simulink model "Lab3_sol"  (R2024a)
settings: Solver=VariableStepAuto  StartTime=0.0  StopTime=10000  MaxStep=0.1  RelTol=1e-3
values from neighbouring files (symbols this model uses):
  A = [-P1 0 -Gb;0 -n 0;0 P3 -P2]    [Bergman_param.m]
  B = [0 1/Vg;1/V1 0;0 0]    [Bergman_param.m]
  Gb = 81    [Bergman_param.m]
  Ib = 15    [Bergman_param.m]
  n = 5/54    (= 0.0925925925926)    [Bergman_param.m]
  p1 = P1    (= 0.003)    [Bergman_param.m]
  p2 = P2    (= 0.025)    [Bergman_param.m]
  p3 = P3    (= 1.3e-05)    [Bergman_param.m]
  V1 = 12    [Bergman_param.m]
undefined symbols (not defined in the file or in its folder): r_, VG
libraries: simulink x4
settings Model: Creator=Diego Regruto  LastModifiedBy=luigi
settings RTWCC: GPUComputeCapability=3.5

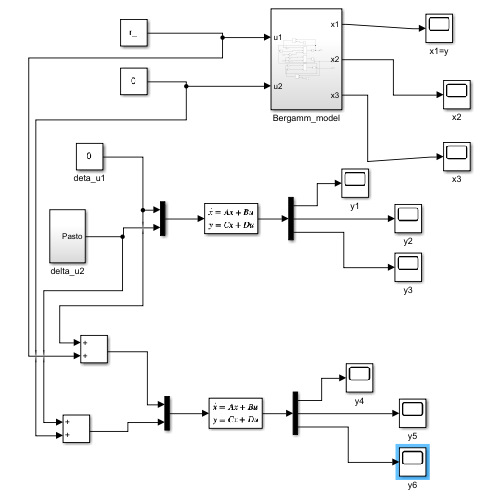
[thumbnail: Simulink's stored preview of the top-level diagram]
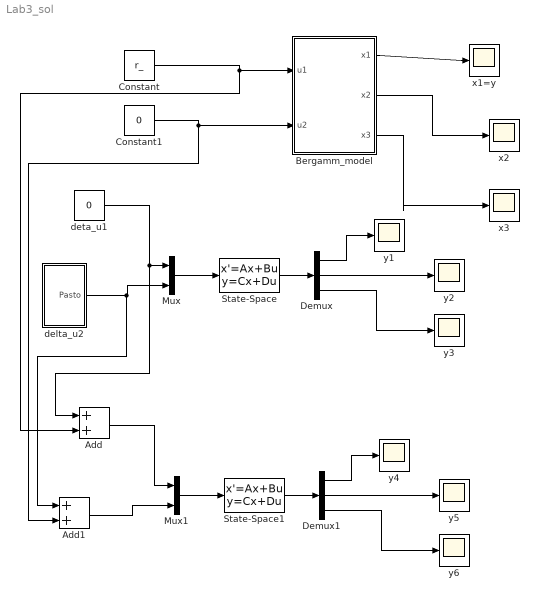
== system Lab3_sol ==
  Add : Sum
  Add1 : Sum
  Bergamm_model : Subsystem
  Constant : Constant  Value=r_
  Constant1 : Constant  Value=0
  Demux : Demux  Outputs=3
  Demux1 : Demux  Outputs=3
  Mux : Mux  Inputs=2
  Mux1 : Mux  Inputs=2
  State-Space : StateSpace  A=A  B=B  C=eye(3,3)  D=zeros(3,2)  InitialCondition=[9 0 0]'
  State-Space1 : StateSpace  A=A  B=B  C=eye(3,3)  D=zeros(3,2)  InitialCondition=[9+81 15 0]'
  delta_u2 : Subsystem
  deta_u1 : Constant  Value=0
  x1=y : Scope
  x2 : Scope
  x3 : Scope
  y{1..6} (6 alike) : Scope
  wires:
  Constant/1 -> Add/2, Bergamm_model/1(u1)
  Constant1/1 -> Add1/2, Bergamm_model/2(u2)
  Bergamm_model/1(x1) -> x1=y/1
  Bergamm_model/2(x2) -> x2/1
  Bergamm_model/3(x3) -> x3/1
  State-Space/1 -> Demux/1
  Mux/1 -> State-Space/1
  Demux/1 -> y1/1
  Demux/2 -> y2/1
  Demux/3 -> y3/1
  delta_u2/1(Pasto) -> Add1/1, Mux/2
  deta_u1/1 -> Add/1, Mux/1
  Demux1/3 -> y6/1
  Mux1/1 -> State-Space1/1
  State-Space1/1 -> Demux1/1
  Demux1/1 -> y4/1
  Add1/1 -> Mux1/2
  Demux1/2 -> y5/1
  Add/1 -> Mux1/1

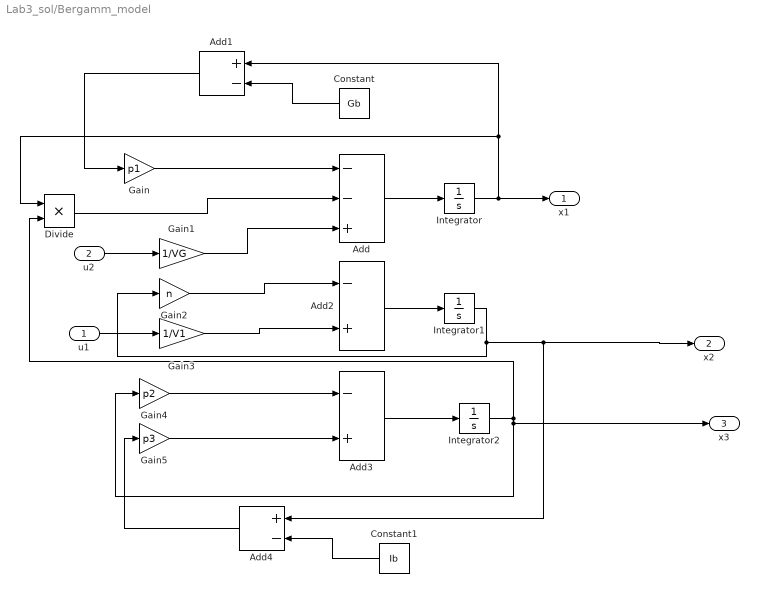
== system Lab3_sol/Bergamm_model ==
  u1 : Inport
  u2 : Inport  Port=2
  Add : Sum  Inputs=--+
  Add1 : Sum  Inputs=+-
  Add2 : Sum  Inputs=-+
  Add3 : Sum  Inputs=-+
  Add4 : Sum  Inputs=+-
  Constant : Constant  Value=Gb
  Constant1 : Constant  Value=Ib
  Divide : Product  Inputs=**
  Gain : Gain  Gain=p1
  Gain1 : Gain  Gain=1/VG
  Gain2 : Gain  Gain=n
  Gain3 : Gain  Gain=1/V1
  Gain4 : Gain  Gain=p2
  Gain5 : Gain  Gain=p3
  Integrator : Integrator
  Integrator1 : Integrator
  Integrator2 : Integrator
  x1 : Outport
  x2 : Outport  Port=2
  x3 : Outport  Port=3
  wires:
  Constant/1 -> Add1/2
  Add4/1 -> Gain5/1
  Divide/1 -> Add/2
  Integrator1/1 -> x2/1, Add4/1, Gain2/1
  Add3/1 -> Integrator2/1
  Constant1/1 -> Add4/2
  Integrator/1 -> x1/1, Divide/1, Add1/1
  Add/1 -> Integrator/1
  Gain4/1 -> Add3/1
  u2/1 -> Gain1/1
  Gain2/1 -> Add2/1
  u1/1 -> Gain3/1
  Add1/1 -> Gain/1
  Gain/1 -> Add/1
  Add2/1 -> Integrator1/1
  Gain3/1 -> Add2/2
  Integrator2/1 -> Divide/2, x3/1, Gain4/1
  Gain5/1 -> Add3/2
  Gain1/1 -> Add/3

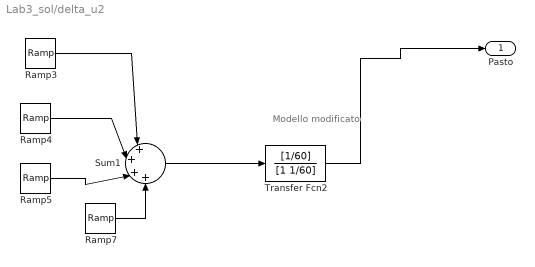
== system Lab3_sol/delta_u2 ==
  note: Modello
      | modificato
  Ramp3 : simulink/Sources/Ramp  slope=12  start=0  InitialOutput=0
  Ramp4 : simulink/Sources/Ramp  slope=-12  start=30  InitialOutput=0
  Ramp5 : simulink/Sources/Ramp  slope=-12  start=90  InitialOutput=0
  Ramp7 : simulink/Sources/Ramp  slope=12  start=120  InitialOutput=0
  Sum1 : Sum  Inputs=|+|+|+|+  InputSameDT=on  SaturateOnIntegerOverflow=on  OutDataTypeStr=Inherit: Same as first input
  Transfer Fcn2 : TransferFcn  Numerator=[1/60]  Denominator=[1 1/60]
  Pasto : Outport
  wires:
  Ramp3/1 -> Sum1/1
  Ramp4/1 -> Sum1/2
  Ramp5/1 -> Sum1/3
  Ramp7/1 -> Sum1/4
  Sum1/1 -> Transfer Fcn2/1
  Transfer Fcn2/1 -> Pasto/1
